simulink model "Cylinder"  (R2014b)
settings: Solver=ode45  StartTime=0.0  StopTime=10.0  RelTol=1e-3
settings Model: Creator=danfa688  LastModifiedBy=danfa688

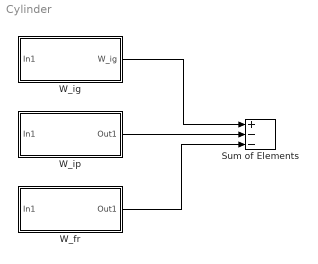
== system Cylinder ==
  Sum of Elements : Sum  Inputs=+--
  W_fr : Subsystem
  W_ig : Subsystem
  W_ip : Subsystem
  wires:
  W_ip/1(Out1) -> Sum of Elements/2
  W_ig/1(W_ig) -> Sum of Elements/1
  W_fr/1(Out1) -> Sum of Elements/3

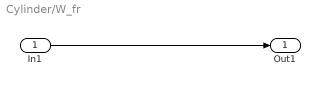
== system Cylinder/W_fr ==
  In1 : Inport
  Out1 : Outport
  wires:
  In1/1 -> Out1/1

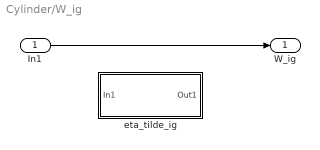
== system Cylinder/W_ig ==
  In1 : Inport
  eta_tilde_ig : Subsystem
  W_ig : Outport
  wires:
  In1/1 -> W_ig/1

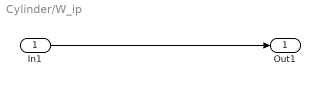
== system Cylinder/W_ip ==
  In1 : Inport
  Out1 : Outport
  wires:
  In1/1 -> Out1/1

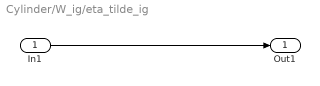
== system Cylinder/W_ig/eta_tilde_ig ==
  In1 : Inport
  Out1 : Outport
  wires:
  In1/1 -> Out1/1
